simulink model "gm_sobelFilter2024a"  (R2024b)
settings: Solver=FixedStepDiscrete  StartTime=0.0  StopTime=2  FixedStep=2.77039007092199e-06  RelTol=1e-3
undefined symbols (not defined in the file or in its folder): gray, R
libraries: hdlsllib x12, visionhdlio x4, visionsources x2
(part 1 of 2)
Description:
  | Sobel Edge Detection Using the MATLAB(R) Function Block
  | This example shows how to use HDL Coder(TM) to check,
  | generate, and verify HDL code for a Sobel Edge Detection
  | block built using the MATLAB Function block.
settings Model: Creator=The MathWorks, Inc.  LastModifiedBy=avate
settings SolverCC: AlgebraicLoopSolver=TrustRegion
settings DataIOCC: LimitDataPoints=on  SaveFormat=Array  SignalLogging=off  ReturnWorkspaceOutputs=off
settings OptimizationCC: BlockReduction=off  ConditionallyExecuteInputs=off  DefaultParameterBehavior=Inlined  ExpressionDepthLimit=2147483647  InitFltsAndDblsToZero=on  EfficientMapNaN2IntZero=off  LifeSpan=inf
settings DebuggingCC: AlgebraicLoopMsg=error  SaveWithParameterizedLinksMsg=none  MergeDetectMultiDrivingBlocksExec=none  SignalResolutionControl=TryResolveAllWithWarning  InheritedTsInSrcMsg=none  MultiTaskDSMMsg=warning  MultiTaskCondExecSysMsg=none  SingleTaskRateTransMsg=error  IntegerOverflowMsg=none  ParameterPrecisionLossMsg=none  FcnCallInpInsideContextMsg=warning  UnconnectedInputMsg=warning  UnconnectedOutputMsg=warning  UnconnectedLineMsg=warning  AllowSymbolicDim=off  StateNameClashWarn=warning  StrictBusMsg=ErrorOnBusTreatedAsVector  SFUnexpectedBacktrackingDiag=warning  SFNoUnconditionalDefaultTransitionDiag=warning  SFExecutionAtInitializationDiag=none  IntegerSaturationMsg=none  ArithmeticOperatorsInVariantConditions=warning
settings HardwareCC: ProdBitPerPointer=32  ProdBitPerSizeT=32  ProdBitPerPtrDiffT=32  ProdLargestAtomicFloat=None  ProdIntDivRoundTo=Undefined  ProdEndianess=Unspecified  ProdWordSize=32  ProdHWDeviceType=ASIC/FPGA  TargetHWDeviceType=32-bit Generic  ProdEqTarget=off
settings ModelReferenceCC: EnableRefExpFcnMdlSchedulingChecks=on  PropagateSignalLabelsOutOfModel=off
settings SFSimCC: SimUseLocalCustomCode=off  CustomCodeUndefinedFunction=UseInterfaceOnly
settings RTWCC: RTWUseLocalCustomCode=off  GPUComputeCapability=3.5  DLArmComputeVersion=19.05
settings CodeAppCC: StateflowObjectComments=on
settings GRTTargetCC: TargetFcnLib=ansi_tfl_tmw.mat  TargetLangStandard=C89/C90 (ANSI)  CombineOutputUpdateFcns=off  GRTInterface=on
settings ConfigComp: CovMetricSettings=dw  CovSaveCumulativeToWorkspaceVar=on  CovSaveSingleToWorkspaceVar=on  CovExternalEMLEnable=off

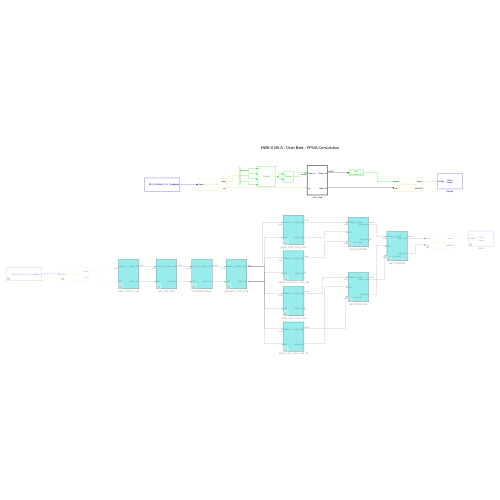
[thumbnail: Simulink's stored preview of the top-level diagram]
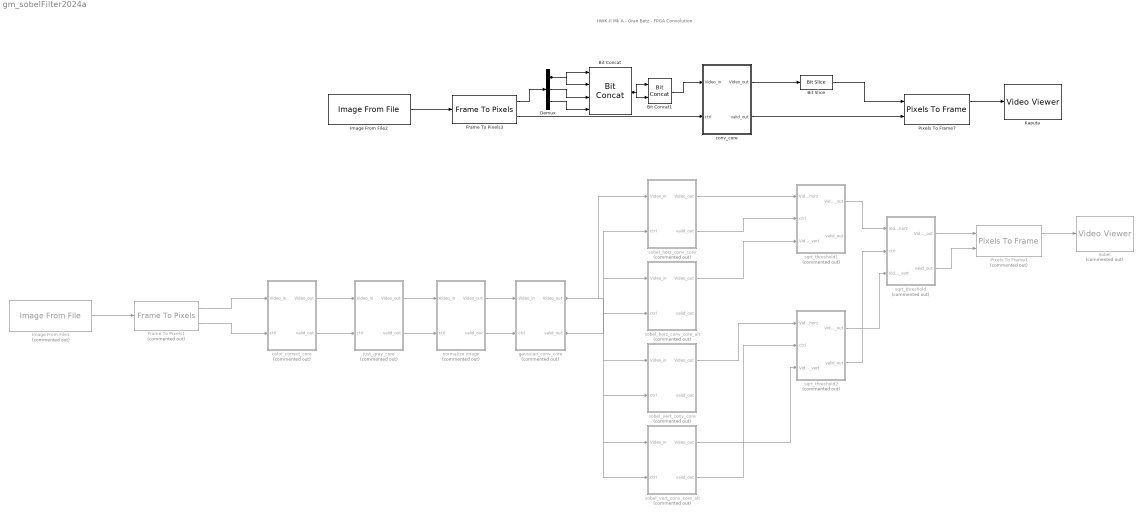
== system gm_sobelFilter2024a ==
  note: HWK-II Mk A - Oran Betz - FPGA Convolution
  Bit Concat : hdlsllib/Logic and Bit Operations/Bit Concat  numInputs=4
  Bit Concat1 : hdlsllib/Logic and Bit Operations/Bit Concat  numInputs=2
  Bit Slice : hdlsllib/Logic and Bit Operations/Bit Slice  lidx=31  ridx=24
  Demux : Demux  Outputs=3
  Frame To Pixels1 : visionhdlio/Frame To Pixels  Commented=on  NumComponents=3  NumPixels=1  VideoFormat=Custom  ActivePixelsPerLine=R  ActiveVideoLines=C  TotalPixelsPerLine=R  TotalVideoLines=C  StartingActiveLine=1  FrontPorch=0  SampleTime=0  VideoFormatCache=Custom  ActivePixelsPerLineCache=R  ActiveVideoLinesCache=C  TotalPixelsPerLineCache=R  TotalVideoLinesCache=C  StartingActiveLineCache=1  FrontPorchCache=0
  Frame To Pixels3 : visionhdlio/Frame To Pixels  NumComponents=3  NumPixels=1  VideoFormat=Custom  ActivePixelsPerLine=R  ActiveVideoLines=C  TotalPixelsPerLine=R  TotalVideoLines=C  StartingActiveLine=1  FrontPorch=0  SampleTime=0  VideoFormatCache=Custom  ActivePixelsPerLineCache=R  ActiveVideoLinesCache=C  TotalPixelsPerLineCache=R  TotalVideoLinesCache=C  StartingActiveLineCache=1  FrontPorchCache=0
  Image From File1 : visionsources/Image From File  Tag=vipblks_nd  Commented=on  FileName=S:\ESD2_Top\ESD2\Final_Proj\Challengers_Sobel\imgs\imgs\BL3_CamLeft_2_5_2.png  Ts=1  imagePorts=One multidimensional signal  OutPortLabels=R|G|B  ImageDataType=Inherit from input image  sdImageDataType=uint(8)  Signed=on  WordLength=16  FractionLengthMode=User-defined  FractionLength=15
  Image From File2 : visionsources/Image From File  Tag=vipblks_nd  FileName=..\imgs\BL3_CamRight_2_5_2.png  Ts=1  imagePorts=One multidimensional signal  OutPortLabels=R|G|B  ImageDataType=Inherit from input image  sdImageDataType=uint(8)  Signed=on  WordLength=16  FractionLengthMode=User-defined  FractionLength=15
  Kaputa : VideoViewer  colormapValue=gray(256)  FigPos=[906 852 825 520]
  Pixels To Frame1 : visionhdlio/Pixels To Frame  Commented=on  NumComponents=1  NumPixels=1  VideoFormat=Custom  ActivePixelsPerLine=R  ActiveVideoLines=C  TotalPixelsPerLine=R  TotalVideoLines=C  VideoFormatCache=Custom  ActivePixelsPerLineCache=R  ActiveVideoLinesCache=C  TotalPixelsPerLineCache=R  TotalVideoLinesCache=C
  Pixels To Frame7 : visionhdlio/Pixels To Frame  NumComponents=1  NumPixels=1  VideoFormat=Custom  ActivePixelsPerLine=R  ActiveVideoLines=C  TotalPixelsPerLine=R  TotalVideoLines=C  VideoFormatCache=Custom  ActivePixelsPerLineCache=R  ActiveVideoLinesCache=C  TotalPixelsPerLineCache=R  TotalVideoLinesCache=C
  Sobel : VideoViewer  Commented=on  colormapValue=gray(256)  FigPos=[2938 790 825 520]
  color_correct_core : Subsystem  Commented=on  TreatAsAtomicUnit=on
  conv_core : Subsystem  TreatAsAtomicUnit=on
  gaussian_conv_core : Subsystem  Commented=on  TreatAsAtomicUnit=on
  just_gray_core : Subsystem  Commented=on  TreatAsAtomicUnit=on
  normalize image : Subsystem  Commented=on  TreatAsAtomicUnit=on
  sobel_horz_conv_core : Subsystem  Commented=on  TreatAsAtomicUnit=on
  sobel_horz_conv_core_alt : Subsystem  Commented=on  TreatAsAtomicUnit=on
  sobel_vert_conv_core : Subsystem  Commented=on  TreatAsAtomicUnit=on
  sobel_vert_conv_core_alt : Subsystem  Commented=on  TreatAsAtomicUnit=on
  sqrt_threshold : Subsystem  Commented=on  TreatAsAtomicUnit=on
  sqrt_threshold1 : Subsystem  Commented=on  TreatAsAtomicUnit=on
  sqrt_threshold2 : Subsystem  Commented=on  TreatAsAtomicUnit=on
  wires:
  Bit Concat/1 -> Bit Concat1/1, Bit Concat1/2
  Bit Concat1/1 -> conv_core/1(Video_in)
  Demux/1 -> Bit Concat/2, Bit Concat/1
  Demux/2 -> Bit Concat/3
  Demux/3 -> Bit Concat/4
  Frame To Pixels1/2 -> color_correct_core/2(ctrl)
  Frame To Pixels1/1 -> color_correct_core/1(Video_in)
  color_correct_core/2(valid_out) -> just_gray_core/2(ctrl)
  color_correct_core/1(Video_out) -> just_gray_core/1(Video_in)
  sobel_vert_conv_core_alt/2(valid_out) -> sqrt_threshold2/2(ctrl)
  sobel_vert_conv_core_alt/1(Video_out) -> sqrt_threshold2/3(Video_in_vert)
  sobel_vert_conv_core/1(Video_out) -> sqrt_threshold2/1(Video_in_horz)
  sobel_horz_conv_core/2(valid_out) -> sqrt_threshold1/2(ctrl)
  sobel_horz_conv_core/1(Video_out) -> sqrt_threshold1/1(Video_in_horz)
  sobel_horz_conv_core_alt/1(Video_out) -> sqrt_threshold1/3(Video_in_vert)
  sqrt_threshold2/2(valid_out) -> sqrt_threshold/2(ctrl)
  sqrt_threshold2/1(Video_out) -> sqrt_threshold/3(Video_in_vert)
  sqrt_threshold1/1(Video_out) -> sqrt_threshold/1(Video_in_horz)
  sqrt_threshold/2(valid_out) -> Pixels To Frame1/2
  sqrt_threshold/1(Video_out) -> Pixels To Frame1/1
  normalize image/2(valid_out) -> gaussian_conv_core/2(ctrl)
  gaussian_conv_core/2(valid_out) -> sobel_horz_conv_core/2(ctrl), sobel_horz_conv_core_alt/2(ctrl), sobel_vert_conv_core_alt/2(ctrl), sobel_vert_conv_core/2(ctrl)
  just_gray_core/1(Video_out) -> normalize image/1(Video_in)
  gaussian_conv_core/1(Video_out) -> sobel_horz_conv_core/1(Video_in), sobel_horz_conv_core_alt/1(Video_in), sobel_vert_conv_core/1(Video_in), sobel_vert_conv_core_alt/1(Video_in)
  just_gray_core/2(valid_out) -> normalize image/2(ctrl)
  normalize image/1(Video_out) -> gaussian_conv_core/1(Video_in)
  Pixels To Frame1/1 -> Sobel/1
  Image From File1/1 -> Frame To Pixels1/1
  Bit Slice/1 -> Pixels To Frame7/1
  conv_core/1(Video_out) -> Bit Slice/1
  conv_core/2(valid_out) -> Pixels To Frame7/2
  Frame To Pixels3/2 -> conv_core/2(ctrl)
  Pixels To Frame7/1 -> Kaputa/1
  Image From File2/1 -> Frame To Pixels3/1
  Frame To Pixels3/1 -> Demux/1

== system gm_sobelFilter2024a/color_correct_core ==
  Video_in : Inport  OutDataTypeStr=uint8
  ctrl : Inport  Port=2
  Bus Selector : BusSelector  OutputSignals=valid
  Subsystem1 : Subsystem
  Video_out : Outport  OutDataTypeStr=uint8  VectorParamsAs1DForOutWhenUnconnected=off
  valid_out : Outport  Port=2  VectorParamsAs1DForOutWhenUnconnected=off
  wires:
  ctrl/1 -> Bus Selector/1, valid_out/1
  Subsystem1/1(Video_out) -> Video_out/1
  Bus Selector/1 -> Subsystem1/Enable  "<valid>"
  Video_in/1 -> Subsystem1/1(channel_in)

== system gm_sobelFilter2024a/conv_core ==
  Video_in : Inport  OutDataTypeStr=fixdt(0, 64, 0)  PortDimensions=1  SampleTime=2.77039007092199e-06
  ctrl : Inport  Port=2
  Bit Concat : hdlsllib/Logic and Bit Operations/Bit Concat  numInputs=8
  Bit Slice : hdlsllib/Logic and Bit Operations/Bit Slice  lidx=double(31)  ridx=double(0)
  color_correct_core : Subsystem
  gaussian_conv_core : Subsystem
  just_gray_core : Subsystem
  normalize image : Subsystem
  sobel_horz_conv_core : Subsystem
  sobel_horz_conv_core_alt : Subsystem
  sobel_vert_conv_core : Subsystem
  sobel_vert_conv_core_alt : Subsystem
  sqrt_threshold : Subsystem
  sqrt_threshold1 : Subsystem
  sqrt_threshold2 : Subsystem
  Video_out : Outport  OutDataTypeStr=uint64  SampleTime=2.77039007092199e-06  VectorParamsAs1DForOutWhenUnconnected=off
  valid_out : Outport  Port=2  VectorParamsAs1DForOutWhenUnconnected=off
  wires:
  normalize image/1(Video_out) -> gaussian_conv_core/1(Video_in)
  Video_in/1 -> Bit Slice/1
  sqrt_threshold1/1(Video_out) -> sqrt_threshold/1(Video_in_horz)
  Bit Slice/1 -> color_correct_core/1(Video_in)
  ctrl/1 -> color_correct_core/2(ctrl)
  color_correct_core/1(Video_out) -> just_gray_core/1(Video_in)
  just_gray_core/2(valid_out) -> normalize image/2(ctrl)
  color_correct_core/2(valid_out) -> just_gray_core/2(ctrl)
  just_gray_core/1(Video_out) -> normalize image/1(Video_in)
  Bit Concat/1 -> Video_out/1
  gaussian_conv_core/2(valid_out) -> sobel_vert_conv_core_alt/2(ctrl), sobel_horz_conv_core_alt/2(ctrl), sobel_vert_conv_core/2(ctrl), sobel_horz_conv_core/2(ctrl)
  normalize image/2(valid_out) -> gaussian_conv_core/2(ctrl)
  gaussian_conv_core/1(Video_out) -> sobel_vert_conv_core/1(Video_in), sobel_vert_conv_core_alt/1(Video_in), sobel_horz_conv_core_alt/1(Video_in), sobel_horz_conv_core/1(Video_in)
  sobel_horz_conv_core/1(Video_out) -> sqrt_threshold1/1(Video_in_horz)
  sobel_horz_conv_core/2(valid_out) -> sqrt_threshold1/2(ctrl)
  sobel_horz_conv_core_alt/1(Video_out) -> sqrt_threshold1/3(Video_in_vert)
  sobel_vert_conv_core/1(Video_out) -> sqrt_threshold2/1(Video_in_horz)
  sobel_vert_conv_core_alt/1(Video_out) -> sqrt_threshold2/3(Video_in_vert)
  sobel_vert_conv_core_alt/2(valid_out) -> sqrt_threshold2/2(ctrl)
  sqrt_threshold2/1(Video_out) -> sqrt_threshold/3(Video_in_vert)
  sqrt_threshold2/2(valid_out) -> sqrt_threshold/2(ctrl)
  sqrt_threshold/1(Video_out) -> Bit Concat/7, Bit Concat/6, Bit Concat/5, Bit Concat/8, Bit Concat/3, Bit Concat/1, Bit Concat/2, Bit Concat/4
  sqrt_threshold/2(valid_out) -> valid_out/1

== system gm_sobelFilter2024a/gaussian_conv_core ==
  note: Coefficients Constants Block
  Video_in : Inport  OutDataTypeStr=uint8
  ctrl : Inport  Port=2
  Bus Selector : BusSelector  OutputSignals=valid
  Constant : Constant  Value=[1/16 1/8 1/16; 1/8 1/4 1/8; 1/16 1/8 1/16];  OutDataTypeStr=fixdt(1,16,12)  SampleTime=-1
  Delay1 : Delay  InitialCondition=0
  Reshape : Reshape
  Subsystem1 : Subsystem
  Transpose : Math  Operator=transpose
  Video_out : Outport  OutDataTypeStr=uint8  VectorParamsAs1DForOutWhenUnconnected=off
  valid_out : Outport  Port=2  VectorParamsAs1DForOutWhenUnconnected=off
  wires:
  Constant/1 -> Transpose/1
  Transpose/1 -> Reshape/1
  Delay1/1 -> valid_out/1
  Reshape/1 -> Subsystem1/2(coeffs)
  Subsystem1/1(Video_out) -> Video_out/1
  Bus Selector/1 -> Subsystem1/Enable  "<valid>"
  ctrl/1 -> Delay1/1, Bus Selector/1
  Video_in/1 -> Subsystem1/1(channel_in)

== system gm_sobelFilter2024a/just_gray_core ==
  Video_in : Inport  OutDataTypeStr=uint8
  ctrl : Inport  Port=2
  Bus Selector : BusSelector  OutputSignals=valid
  Subsystem1 : Subsystem
  Video_out : Outport  OutDataTypeStr=uint8  VectorParamsAs1DForOutWhenUnconnected=off
  valid_out : Outport  Port=2  VectorParamsAs1DForOutWhenUnconnected=off
  wires:
  ctrl/1 -> Bus Selector/1, valid_out/1
  Subsystem1/1(Video_out) -> Video_out/1
  Bus Selector/1 -> Subsystem1/Enable  "<valid>"
  Video_in/1 -> Subsystem1/1(channel_in)

== system gm_sobelFilter2024a/normalize image ==
  Video_in : Inport  OutDataTypeStr=uint8
  ctrl : Inport  Port=2
  Bus Selector : BusSelector  OutputSignals=valid
  Delay3 : Delay  DelayLength=4  InitialCondition=0
  Subsystem1 : Subsystem
  Video_out : Outport  OutDataTypeStr=uint8  VectorParamsAs1DForOutWhenUnconnected=off
  valid_out : Outport  Port=2  VectorParamsAs1DForOutWhenUnconnected=off
  wires:
  Delay3/1 -> valid_out/1
  ctrl/1 -> Bus Selector/1, Delay3/1
  Subsystem1/1(Video_out) -> Video_out/1
  Bus Selector/1 -> Subsystem1/Enable  "<valid>"
  Video_in/1 -> Subsystem1/1(channel_in)

== system gm_sobelFilter2024a/sobel_horz_conv_core ==
  note: Coefficients Constants Block
  Video_in : Inport  OutDataTypeStr=uint8
  ctrl : Inport  Port=2
  Bus Selector : BusSelector  OutputSignals=valid
  Constant : Constant  Value=[1 0 -1; 2 0 -2; 1 0 -1];  OutDataTypeStr=fixdt(1,16,12)  SampleTime=-1
  Delay1 : Delay  InitialCondition=0
  Reshape : Reshape
  Subsystem1 : Subsystem
  Transpose : Math  Operator=transpose
  Video_out : Outport  OutDataTypeStr=uint8  VectorParamsAs1DForOutWhenUnconnected=off
  valid_out : Outport  Port=2  VectorParamsAs1DForOutWhenUnconnected=off
  wires:
  Constant/1 -> Transpose/1
  Transpose/1 -> Reshape/1
  Delay1/1 -> valid_out/1
  Reshape/1 -> Subsystem1/2(coeffs)
  Subsystem1/1(Video_out) -> Video_out/1
  Bus Selector/1 -> Subsystem1/Enable  "<valid>"
  ctrl/1 -> Delay1/1, Bus Selector/1
  Video_in/1 -> Subsystem1/1(channel_in)

== system gm_sobelFilter2024a/sobel_horz_conv_core_alt ==
  note: Coefficients Constants Block
  Video_in : Inport  OutDataTypeStr=uint8
  ctrl : Inport  Port=2
  Bus Selector : BusSelector  OutputSignals=valid
  Constant : Constant  Value=[-1 0 1; -2 0 2; -1 0 1];  OutDataTypeStr=fixdt(1,16,12)  SampleTime=-1
  Delay1 : Delay  InitialCondition=0
  Reshape : Reshape
  Subsystem1 : Subsystem
  Transpose : Math  Operator=transpose
  Video_out : Outport  OutDataTypeStr=uint8  VectorParamsAs1DForOutWhenUnconnected=off
  valid_out : Outport  Port=2  VectorParamsAs1DForOutWhenUnconnected=off
  wires:
  Constant/1 -> Transpose/1
  Transpose/1 -> Reshape/1
  Delay1/1 -> valid_out/1
  Reshape/1 -> Subsystem1/2(coeffs)
  Subsystem1/1(Video_out) -> Video_out/1
  Bus Selector/1 -> Subsystem1/Enable  "<valid>"
  ctrl/1 -> Delay1/1, Bus Selector/1
  Video_in/1 -> Subsystem1/1(channel_in)

== system gm_sobelFilter2024a/sobel_vert_conv_core ==
  note: Coefficients Constants Block
  Video_in : Inport  OutDataTypeStr=uint8
  ctrl : Inport  Port=2
  Bus Selector : BusSelector  OutputSignals=valid
  Constant : Constant  Value=|  OutDataTypeStr=fixdt(1,16,12)  SampleTime=-1
      | [1 2 1;  0 0 0;
      | -1 -2 -1];
  Delay1 : Delay  InitialCondition=0
  Reshape : Reshape
  Subsystem1 : Subsystem
  Transpose : Math  Operator=transpose
  Video_out : Outport  OutDataTypeStr=uint8  VectorParamsAs1DForOutWhenUnconnected=off
  valid_out : Outport  Port=2  VectorParamsAs1DForOutWhenUnconnected=off
  wires:
  Constant/1 -> Transpose/1
  Transpose/1 -> Reshape/1
  Delay1/1 -> valid_out/1
  Reshape/1 -> Subsystem1/2(coeffs)
  Subsystem1/1(Video_out) -> Video_out/1
  Bus Selector/1 -> Subsystem1/Enable  "<valid>"
  ctrl/1 -> Delay1/1, Bus Selector/1
  Video_in/1 -> Subsystem1/1(channel_in)

== system gm_sobelFilter2024a/sobel_vert_conv_core_alt ==
  note: Coefficients Constants Block
  Video_in : Inport  OutDataTypeStr=uint8
  ctrl : Inport  Port=2
  Bus Selector : BusSelector  OutputSignals=valid
  Constant : Constant  Value=|  OutDataTypeStr=fixdt(1,16,12)  SampleTime=-1
      | [-1 -2 -1;  0 0 0;
      | 1 2 1];
  Delay1 : Delay  InitialCondition=0
  Reshape : Reshape
  Subsystem1 : Subsystem
  Transpose : Math  Operator=transpose
  Video_out : Outport  OutDataTypeStr=uint8  VectorParamsAs1DForOutWhenUnconnected=off
  valid_out : Outport  Port=2  VectorParamsAs1DForOutWhenUnconnected=off
  wires:
  Constant/1 -> Transpose/1
  Transpose/1 -> Reshape/1
  Delay1/1 -> valid_out/1
  Reshape/1 -> Subsystem1/2(coeffs)
  Subsystem1/1(Video_out) -> Video_out/1
  Bus Selector/1 -> Subsystem1/Enable  "<valid>"
  ctrl/1 -> Delay1/1, Bus Selector/1
  Video_in/1 -> Subsystem1/1(channel_in)

== system gm_sobelFilter2024a/sqrt_threshold ==
  note: Coefficients Constants Block
  Video_in_horz : Inport  OutDataTypeStr=uint8
  ctrl : Inport  Port=2
  Video_in_vert : Inport  Port=3  OutDataTypeStr=uint8
  Bus Selector : BusSelector  OutputSignals=valid
  Constant : Constant  Value=|  OutDataTypeStr=fixdt(1,16,12)  SampleTime=-1
      | [1 2 1;  0 0 0;
      | -1 -2 -2];
  Delay1 : Delay  DelayLength=4  InitialCondition=0
  Reshape : Reshape
  Subsystem2 : Subsystem
  Transpose : Math  Operator=transpose
  Video_out : Outport  OutDataTypeStr=uint8  VectorParamsAs1DForOutWhenUnconnected=off
  valid_out : Outport  Port=2  VectorParamsAs1DForOutWhenUnconnected=off
  wires:
  Video_in_vert/1 -> Subsystem2/2(channel_in_vert)
  Constant/1 -> Transpose/1
  Transpose/1 -> Reshape/1
  Delay1/1 -> valid_out/1
  Reshape/1 -> Subsystem2/3(coeffs)
  Subsystem2/1(Video_out) -> Video_out/1
  Bus Selector/1 -> Subsystem2/Enable  "<valid>"
  ctrl/1 -> Delay1/1, Bus Selector/1
  Video_in_horz/1 -> Subsystem2/1(channel_horz)

== system gm_sobelFilter2024a/sqrt_threshold1 ==
  note: Coefficients Constants Block
  Video_in_horz : Inport  OutDataTypeStr=uint8
  ctrl : Inport  Port=2
  Video_in_vert : Inport  Port=3  OutDataTypeStr=uint8
  Bus Selector : BusSelector  OutputSignals=valid
  Constant : Constant  Value=|  OutDataTypeStr=fixdt(1,16,12)  SampleTime=-1
      | [1 2 1;  0 0 0;
      | -1 -2 -2];
  Delay1 : Delay  DelayLength=4  InitialCondition=0
  Reshape : Reshape
  Subsystem2 : Subsystem
  Transpose : Math  Operator=transpose
  Video_out : Outport  OutDataTypeStr=uint8  VectorParamsAs1DForOutWhenUnconnected=off
  valid_out : Outport  Port=2  VectorParamsAs1DForOutWhenUnconnected=off
  wires:
  Video_in_vert/1 -> Subsystem2/2(channel_in_vert)
  Constant/1 -> Transpose/1
  Transpose/1 -> Reshape/1
  Delay1/1 -> valid_out/1
  Reshape/1 -> Subsystem2/3(coeffs)
  Subsystem2/1(Video_out) -> Video_out/1
  Bus Selector/1 -> Subsystem2/Enable  "<valid>"
  ctrl/1 -> Delay1/1, Bus Selector/1
  Video_in_horz/1 -> Subsystem2/1(channel_horz)

== system gm_sobelFilter2024a/sqrt_threshold2 ==
  note: Coefficients Constants Block
  Video_in_horz : Inport  OutDataTypeStr=uint8
  ctrl : Inport  Port=2
  Video_in_vert : Inport  Port=3  OutDataTypeStr=uint8
  Bus Selector : BusSelector  OutputSignals=valid
  Constant : Constant  Value=|  OutDataTypeStr=fixdt(1,16,12)  SampleTime=-1
      | [1 2 1;  0 0 0;
      | -1 -2 -2];
  Delay1 : Delay  DelayLength=4  InitialCondition=0
  Reshape : Reshape
  Subsystem2 : Subsystem
  Transpose : Math  Operator=transpose
  Video_out : Outport  OutDataTypeStr=uint8  VectorParamsAs1DForOutWhenUnconnected=off
  valid_out : Outport  Port=2  VectorParamsAs1DForOutWhenUnconnected=off
  wires:
  Video_in_vert/1 -> Subsystem2/2(channel_in_vert)
  Constant/1 -> Transpose/1
  Transpose/1 -> Reshape/1
  Delay1/1 -> valid_out/1
  Reshape/1 -> Subsystem2/3(coeffs)
  Subsystem2/1(Video_out) -> Video_out/1
  Bus Selector/1 -> Subsystem2/Enable  "<valid>"
  ctrl/1 -> Delay1/1, Bus Selector/1
  Video_in_horz/1 -> Subsystem2/1(channel_horz)

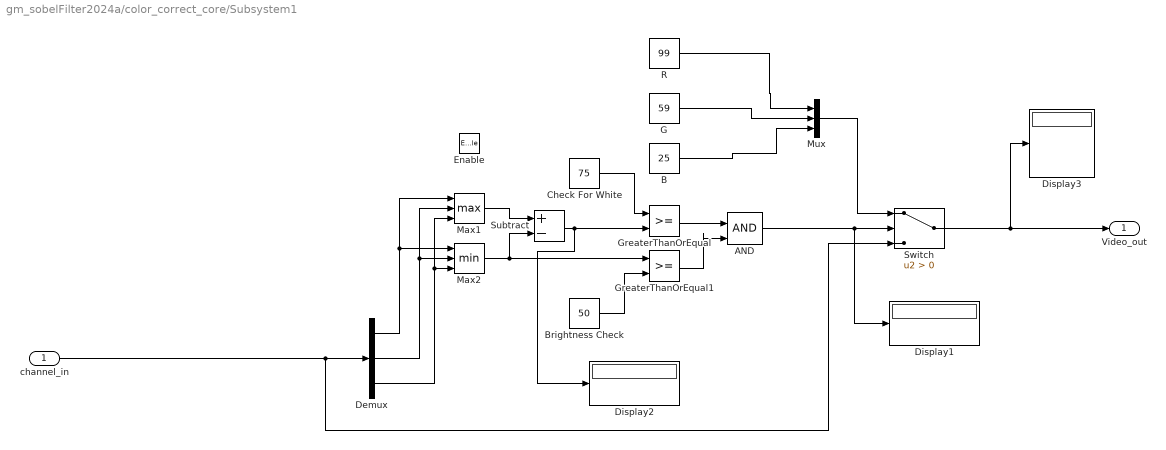
== system gm_sobelFilter2024a/color_correct_core/Subsystem1 ==
  channel_in : Inport  OutDataTypeStr=uint8
  Enable : EnablePort
  AND : Logic  IconShape=distinctive  AllPortsSameDT=off  OutDataTypeStr=boolean
  B : Constant  Value=25  OutDataTypeStr=uint8
  Brightness Check : Constant  Value=50  OutDataTypeStr=uint8
  Check For White : Constant  Value=75  OutDataTypeStr=uint8
  Demux : Demux  Outputs=3
  Display1 : Display
      settings: Format=binary (Stored Integer)
  Display2 : Display
      settings: Format=binary (Stored Integer)
  Display3 : Display
      settings: Format=binary (Stored Integer)
  G : Constant  Value=59  OutDataTypeStr=uint8
  GreaterThanOrEqual : RelationalOperator  OutDataTypeStr=boolean  RndMeth=Simplest  InputSameDT=off
  GreaterThanOrEqual1 : RelationalOperator  OutDataTypeStr=boolean  RndMeth=Simplest  InputSameDT=off
  Max1 : MinMax  Function=max  Inputs=3
  Max2 : MinMax  Inputs=3
  Mux : Mux  Inputs=3
  R : Constant  Value=99  OutDataTypeStr=uint8
  Subtract : Sum  Inputs=+-
  Switch : Switch  Criteria=u2 > Threshold  SaturateOnIntegerOverflow=off  InputSameDT=off
  Video_out : Outport  OutDataTypeStr=uint8  InitialOutput=[0]
  wires:
  Mux/1 -> Switch/1
  Switch/1 -> Video_out/1, Display3/1
  B/1 -> Mux/3
  G/1 -> Mux/2
  R/1 -> Mux/1
  AND/1 -> Switch/2, Display1/1
  Subtract/1 -> Display2/1, GreaterThanOrEqual/2
  GreaterThanOrEqual1/1 -> AND/2
  Brightness Check/1 -> GreaterThanOrEqual1/2
  GreaterThanOrEqual/1 -> AND/1
  Check For White/1 -> GreaterThanOrEqual/1
  Max2/1 -> Subtract/2, GreaterThanOrEqual1/1
  Max1/1 -> Subtract/1
  Demux/2 -> Max1/2, Max2/2
  Demux/1 -> Max1/1, Max2/1
  channel_in/1 -> Demux/1, Switch/3
  Demux/3 -> Max1/3, Max2/3

== system gm_sobelFilter2024a/conv_core/color_correct_core ==
  Video_in : Inport  OutDataTypeStr=uint32  PortDimensions=1  SampleTime=2.77039007092199e-06
  ctrl : Inport  Port=2
  Subsystem1 : Subsystem
  bus_selector : BusSelector  OutputSignals=valid
  Video_out : Outport  OutDataTypeStr=uint32  SampleTime=2.77039007092199e-06  VectorParamsAs1DForOutWhenUnconnected=off
  valid_out : Outport  Port=2  VectorParamsAs1DForOutWhenUnconnected=off
  wires:
  ctrl/1 -> bus_selector/1, valid_out/1
  bus_selector/1 -> Subsystem1/Enable  "<valid>"
  Video_in/1 -> Subsystem1/1(channel_in)
  Subsystem1/1(Video_out) -> Video_out/1

== system gm_sobelFilter2024a/conv_core/gaussian_conv_core ==
  note: Coefficients Constants Block
  Video_in : Inport  OutDataTypeStr=uint8  PortDimensions=1  SampleTime=2.77039007092199e-06
  ctrl : Inport  Port=2
  Constant : Constant  Value=[0.0625;0.125;0.0625;0.125;0.25;0.125;0.0625;0.125;0.0625]  OutDataTypeStr=fixdt(1, 16, 12)  SampleTime=2.77039007092199e-06
  Delay1 : Delay  DelayLength=double(2)  InitialCondition=0  SampleTime=2.77039007092199e-06
  Reshape : Reshape  OutputDimensions=[9]
  Subsystem1 : Subsystem
  Transpose : Math  Operator=transpose  OutDataTypeStr=fixdt(1, 16, 12)
  bus_selector : BusSelector  OutputSignals=valid
  t : Reshape  OutputDimensionality=Customize  OutputDimensions=[3,3]
  Video_out : Outport  OutDataTypeStr=uint8  SampleTime=2.77039007092199e-06  VectorParamsAs1DForOutWhenUnconnected=off
  valid_out : Outport  Port=2  VectorParamsAs1DForOutWhenUnconnected=off
  wires:
  Constant/1 -> t/1
  Reshape/1 -> Subsystem1/2(coeffs)
  t/1 -> Transpose/1
  Transpose/1 -> Reshape/1
  bus_selector/1 -> Subsystem1/Enable  "<valid>"
  Delay1/1 -> valid_out/1
  ctrl/1 -> bus_selector/1, Delay1/1
  Video_in/1 -> Subsystem1/1(channel_in)
  Subsystem1/1(Video_out) -> Video_out/1

== system gm_sobelFilter2024a/conv_core/just_gray_core ==
  Video_in : Inport  OutDataTypeStr=uint32  PortDimensions=1  SampleTime=2.77039007092199e-06
  ctrl : Inport  Port=2
  Subsystem1 : Subsystem
  bus_selector : BusSelector  OutputSignals=valid
  Video_out : Outport  OutDataTypeStr=uint8  SampleTime=2.77039007092199e-06  VectorParamsAs1DForOutWhenUnconnected=off
  valid_out : Outport  Port=2  VectorParamsAs1DForOutWhenUnconnected=off
  wires:
  ctrl/1 -> bus_selector/1, valid_out/1
  bus_selector/1 -> Subsystem1/Enable  "<valid>"
  Subsystem1/1(Video_out) -> Video_out/1
  Video_in/1 -> Subsystem1/1(channel_in)

== system gm_sobelFilter2024a/conv_core/normalize image ==
  Video_in : Inport  OutDataTypeStr=uint8  PortDimensions=1  SampleTime=2.77039007092199e-06
  ctrl : Inport  Port=2
  Delay3 : Delay  DelayLength=double(4)  InitialCondition=0  SampleTime=2.77039007092199e-06
  Subsystem1 : Subsystem
  bus_selector : BusSelector  OutputSignals=valid
  Video_out : Outport  OutDataTypeStr=uint8  SampleTime=2.77039007092199e-06  VectorParamsAs1DForOutWhenUnconnected=off
  valid_out : Outport  Port=2  VectorParamsAs1DForOutWhenUnconnected=off
  wires:
  Subsystem1/1(Video_out) -> Video_out/1
  Delay3/1 -> valid_out/1
  ctrl/1 -> bus_selector/1, Delay3/1
  bus_selector/1 -> Subsystem1/Enable  "<valid>"
  Video_in/1 -> Subsystem1/1(channel_in)

== system gm_sobelFilter2024a/conv_core/sobel_horz_conv_core ==
  note: Coefficients Constants Block
  Video_in : Inport  OutDataTypeStr=uint8  PortDimensions=1  SampleTime=2.77039007092199e-06
  ctrl : Inport  Port=2
  Constant : Constant  Value=[1;2;1;0;0;0;-1;-2;-1]  OutDataTypeStr=fixdt(1, 16, 12)  SampleTime=2.77039007092199e-06
  Delay1 : Delay  DelayLength=double(2)  InitialCondition=0  SampleTime=2.77039007092199e-06
  Reshape : Reshape  OutputDimensions=[9]
  Subsystem1 : Subsystem
  Transpose : Math  Operator=transpose  OutDataTypeStr=fixdt(1, 16, 12)
  bus_selector : BusSelector  OutputSignals=valid
  t : Reshape  OutputDimensionality=Customize  OutputDimensions=[3,3]
  Video_out : Outport  OutDataTypeStr=uint8  SampleTime=2.77039007092199e-06  VectorParamsAs1DForOutWhenUnconnected=off
  valid_out : Outport  Port=2  VectorParamsAs1DForOutWhenUnconnected=off
  wires:
  Reshape/1 -> Subsystem1/2(coeffs)
  t/1 -> Transpose/1
  bus_selector/1 -> Subsystem1/Enable  "<valid>"
  ctrl/1 -> bus_selector/1, Delay1/1
  Constant/1 -> t/1
  Transpose/1 -> Reshape/1
  Video_in/1 -> Subsystem1/1(channel_in)
  Delay1/1 -> valid_out/1
  Subsystem1/1(Video_out) -> Video_out/1

== system gm_sobelFilter2024a/conv_core/sobel_horz_conv_core_alt ==
  note: Coefficients Constants Block
  Video_in : Inport  OutDataTypeStr=uint8  PortDimensions=1  SampleTime=2.77039007092199e-06
  ctrl : Inport  Port=2
  Constant : Constant  Value=[-1;-2;-1;0;0;0;1;2;1]  OutDataTypeStr=fixdt(1, 16, 12)  SampleTime=2.77039007092199e-06
  Reshape : Reshape  OutputDimensions=[9]
  Subsystem1 : Subsystem
  Transpose : Math  Operator=transpose  OutDataTypeStr=fixdt(1, 16, 12)
  bus_selector : BusSelector  OutputSignals=valid
  t : Reshape  OutputDimensionality=Customize  OutputDimensions=[3,3]
  Video_out : Outport  OutDataTypeStr=uint8  SampleTime=2.77039007092199e-06  VectorParamsAs1DForOutWhenUnconnected=off
  wires:
  Video_in/1 -> Subsystem1/1(channel_in)
  Constant/1 -> t/1
  Transpose/1 -> Reshape/1
  t/1 -> Transpose/1
  Reshape/1 -> Subsystem1/2(coeffs)
  bus_selector/1 -> Subsystem1/Enable  "<valid>"
  ctrl/1 -> bus_selector/1
  Subsystem1/1(Video_out) -> Video_out/1

== system gm_sobelFilter2024a/conv_core/sobel_vert_conv_core ==
  note: Coefficients Constants Block
  Video_in : Inport  OutDataTypeStr=uint8  PortDimensions=1  SampleTime=2.77039007092199e-06
  ctrl : Inport  Port=2
  Constant : Constant  Value=[1;0;-1;2;0;-2;1;0;-1]  OutDataTypeStr=fixdt(1, 16, 12)  SampleTime=2.77039007092199e-06
  Reshape : Reshape  OutputDimensions=[9]
  Subsystem1 : Subsystem
  Transpose : Math  Operator=transpose  OutDataTypeStr=fixdt(1, 16, 12)
  bus_selector : BusSelector  OutputSignals=valid
  t : Reshape  OutputDimensionality=Customize  OutputDimensions=[3,3]
  Video_out : Outport  OutDataTypeStr=uint8  SampleTime=2.77039007092199e-06  VectorParamsAs1DForOutWhenUnconnected=off
  wires:
  Reshape/1 -> Subsystem1/2(coeffs)
  bus_selector/1 -> Subsystem1/Enable  "<valid>"
  t/1 -> Transpose/1
  Constant/1 -> t/1
  Subsystem1/1(Video_out) -> Video_out/1
  Video_in/1 -> Subsystem1/1(channel_in)
  ctrl/1 -> bus_selector/1
  Transpose/1 -> Reshape/1

== system gm_sobelFilter2024a/conv_core/sobel_vert_conv_core_alt ==
  note: Coefficients Constants Block
  Video_in : Inport  OutDataTypeStr=uint8  PortDimensions=1  SampleTime=2.77039007092199e-06
  ctrl : Inport  Port=2
  Constant : Constant  Value=[-1;0;1;-2;0;2;-1;0;1]  OutDataTypeStr=fixdt(1, 16, 12)  SampleTime=2.77039007092199e-06
  Delay1 : Delay  DelayLength=double(2)  InitialCondition=0  SampleTime=2.77039007092199e-06
  Reshape : Reshape  OutputDimensions=[9]
  Subsystem1 : Subsystem
  Transpose : Math  Operator=transpose  OutDataTypeStr=fixdt(1, 16, 12)
  bus_selector : BusSelector  OutputSignals=valid
  t : Reshape  OutputDimensionality=Customize  OutputDimensions=[3,3]
  Video_out : Outport  OutDataTypeStr=uint8  SampleTime=2.77039007092199e-06  VectorParamsAs1DForOutWhenUnconnected=off
  valid_out : Outport  Port=2  VectorParamsAs1DForOutWhenUnconnected=off
  wires:
  Constant/1 -> t/1
  Reshape/1 -> Subsystem1/2(coeffs)
  Transpose/1 -> Reshape/1
  t/1 -> Transpose/1
  ctrl/1 -> bus_selector/1, Delay1/1
  bus_selector/1 -> Subsystem1/Enable  "<valid>"
  Delay1/1 -> valid_out/1
  Video_in/1 -> Subsystem1/1(channel_in)
  Subsystem1/1(Video_out) -> Video_out/1

== system gm_sobelFilter2024a/conv_core/sqrt_threshold ==
  note: Coefficients Constants Block
  Video_in_horz : Inport  OutDataTypeStr=uint8  PortDimensions=1  SampleTime=2.77039007092199e-06
  ctrl : Inport  Port=2
  Video_in_vert : Inport  Port=3  OutDataTypeStr=uint8  PortDimensions=1  SampleTime=2.77039007092199e-06
  Delay1 : Delay  DelayLength=double(4)  InitialCondition=0  SampleTime=2.77039007092199e-06
  Subsystem2 : Subsystem
  bus_selector : BusSelector  OutputSignals=valid
  Video_out : Outport  OutDataTypeStr=uint8  SampleTime=2.77039007092199e-06  VectorParamsAs1DForOutWhenUnconnected=off
  valid_out : Outport  Port=2  VectorParamsAs1DForOutWhenUnconnected=off
  wires:
  bus_selector/1 -> Subsystem2/Enable  "<valid>"
  ctrl/1 -> bus_selector/1, Delay1/1
  Delay1/1 -> valid_out/1
  Video_in_horz/1 -> Subsystem2/1(channel_horz)
  Video_in_vert/1 -> Subsystem2/2(channel_in_vert)
  Subsystem2/1(Video_out) -> Video_out/1

== system gm_sobelFilter2024a/conv_core/sqrt_threshold1 ==
  note: Coefficients Constants Block
  Video_in_horz : Inport  OutDataTypeStr=uint8  PortDimensions=1  SampleTime=2.77039007092199e-06
  ctrl : Inport  Port=2
  Video_in_vert : Inport  Port=3  OutDataTypeStr=uint8  PortDimensions=1  SampleTime=2.77039007092199e-06
  Delay1 : Delay  DelayLength=double(4)  InitialCondition=0  SampleTime=2.77039007092199e-06
  Subsystem2 : Subsystem
  bus_selector : BusSelector  OutputSignals=valid
  Video_out : Outport  OutDataTypeStr=uint8  SampleTime=2.77039007092199e-06  VectorParamsAs1DForOutWhenUnconnected=off
  valid_out : Outport  Port=2  VectorParamsAs1DForOutWhenUnconnected=off
  wires:
  Subsystem2/1(Video_out) -> Video_out/1
  Video_in_vert/1 -> Subsystem2/2(channel_in_vert)
  Video_in_horz/1 -> Subsystem2/1(channel_horz)
  Delay1/1 -> valid_out/1
  ctrl/1 -> Delay1/1, bus_selector/1
  bus_selector/1 -> Subsystem2/Enable  "<valid>"

== system gm_sobelFilter2024a/conv_core/sqrt_threshold2 ==
  note: Coefficients Constants Block
  Video_in_horz : Inport  OutDataTypeStr=uint8  PortDimensions=1  SampleTime=2.77039007092199e-06
  ctrl : Inport  Port=2
  Video_in_vert : Inport  Port=3  OutDataTypeStr=uint8  PortDimensions=1  SampleTime=2.77039007092199e-06
  Delay1 : Delay  DelayLength=double(4)  InitialCondition=0  SampleTime=2.77039007092199e-06
  Subsystem2 : Subsystem
  bus_selector : BusSelector  OutputSignals=valid
  Video_out : Outport  OutDataTypeStr=uint8  SampleTime=2.77039007092199e-06  VectorParamsAs1DForOutWhenUnconnected=off
  valid_out : Outport  Port=2  VectorParamsAs1DForOutWhenUnconnected=off
  wires:
  Subsystem2/1(Video_out) -> Video_out/1
  Video_in_vert/1 -> Subsystem2/2(channel_in_vert)
  Video_in_horz/1 -> Subsystem2/1(channel_horz)
  Delay1/1 -> valid_out/1
  ctrl/1 -> Delay1/1, bus_selector/1
  bus_selector/1 -> Subsystem2/Enable  "<valid>"

== system gm_sobelFilter2024a/gaussian_conv_core/Subsystem1 ==
  note: slice out gray
  channel_in : Inport  OutDataTypeStr=uint8
  coeffs : Inport  Port=2
  Enable : EnablePort
  Delay1 : Delay  DelayLength=1  InitialCondition=0
  Delay2 : Delay  DelayLength=1  InitialCondition=0
  Display : Display
      settings: Format=hex (Stored Integer)
  Mux : Mux  Inputs=9
  Product : Product  SaturateOnIntegerOverflow=on
  Sum of Elements : Sum  Inputs=+  OutDataTypeStr=uint8  SaturateOnIntegerOverflow=on
  slicer : Subsystem
  Video_out : Outport  OutDataTypeStr=uint8  InitialOutput=[0]
  wires:
  Delay2/1 -> Video_out/1
  Sum of Elements/1 -> Delay2/1
  Delay1/1 -> Sum of Elements/1
  Product/1 -> Delay1/1
  coeffs/1 -> Display/1, Product/1
  Mux/1 -> Product/2
  slicer/8(out_8) -> Mux/8
  channel_in/1 -> slicer/1(channel_in)
  slicer/2(out_2) -> Mux/2
  slicer/4(out_4) -> Mux/4
  slicer/6(out_6) -> Mux/6
  slicer/3(out_3) -> Mux/3
  slicer/7(out_7) -> Mux/7
  slicer/5(out_5) -> Mux/5
  slicer/9(out_9) -> Mux/9
  slicer/1(out_1) -> Mux/1

== system gm_sobelFilter2024a/just_gray_core/Subsystem1 ==
  note: Grayscale = (R * 0.25) + (G * 0.5) + (B * 0.0625)
  note: slice out gray
  channel_in : Inport  OutDataTypeStr=uint8
  Enable : EnablePort
  Demux : Demux  Outputs=3
  Shift Arithmetic3 : ArithShift  BitShiftNumber=1  BitShiftDirection=Right
  Shift Arithmetic4 : ArithShift  BitShiftNumber=2  BitShiftDirection=Right
  Shift Arithmetic5 : ArithShift  BitShiftNumber=4  BitShiftDirection=Right
  Sum : Sum  Inputs=+++  OutDataTypeStr=uint8
  Video_out : Outport  OutDataTypeStr=uint8  InitialOutput=[0]
  wires:
  Shift Arithmetic5/1 -> Sum/3
  Shift Arithmetic3/1 -> Sum/2
  Demux/1 -> Shift Arithmetic4/1
  Demux/2 -> Shift Arithmetic3/1
  Shift Arithmetic4/1 -> Sum/1
  channel_in/1 -> Demux/1
  Demux/3 -> Shift Arithmetic5/1
  Sum/1 -> Video_out/1

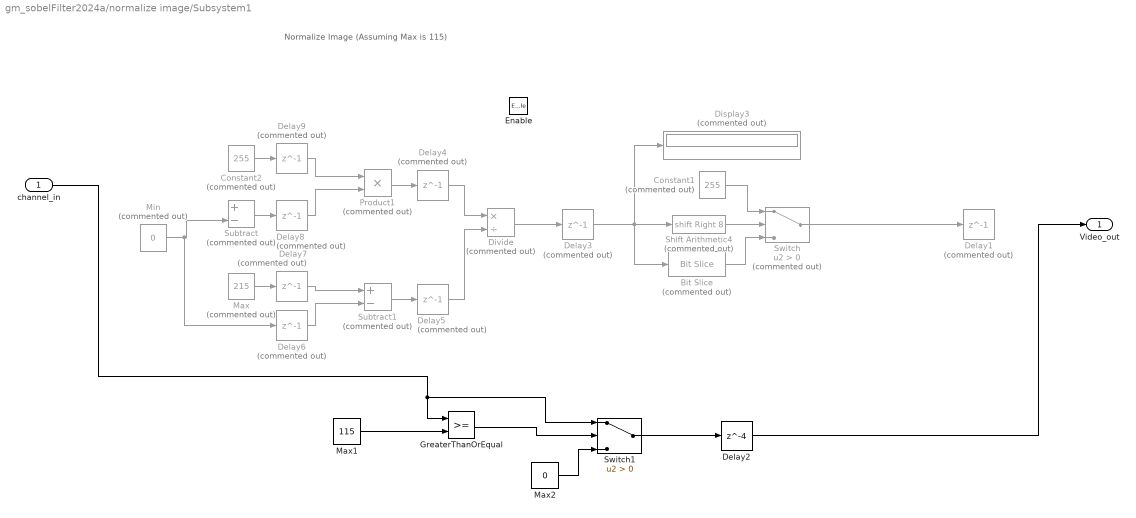
== system gm_sobelFilter2024a/normalize image/Subsystem1 ==
  note: Normalize Image (Assuming Max is 115)
  channel_in : Inport  OutDataTypeStr=uint8
  Enable : EnablePort
  Bit Slice : hdlsllib/Logic and Bit Operations/Bit Slice  Commented=on  lidx=7  ridx=0
  Constant1 : Constant  Commented=on  Value=255  OutDataTypeStr=uint8
  Constant2 : Constant  Commented=on  Value=255  OutDataTypeStr=uint8
  Delay{1,3..9} (8 alike) : Delay  Commented=on  DelayLength=1  InitialCondition=0
  Delay2 : Delay  DelayLength=4  InitialCondition=0
  Display3 : Display  Commented=on
      settings: Format=binary (Stored Integer)
  Divide : Product  Commented=on  Inputs=*/
  GreaterThanOrEqual : RelationalOperator  OutDataTypeStr=boolean  RndMeth=Simplest  InputSameDT=off
  Max : Constant  Commented=on  Value=215  OutDataTypeStr=uint8
  Max1 : Constant  Value=115  OutDataTypeStr=uint8
  Max2 : Constant  Value=0  OutDataTypeStr=uint8
  Min : Constant  Commented=on  Value=0  OutDataTypeStr=uint8
  Product1 : Product  Commented=on  SaturateOnIntegerOverflow=on
  Shift Arithmetic4 : ArithShift  Commented=on  BitShiftNumber=8  BitShiftDirection=Right
  Subtract : Sum  Commented=on  Inputs=+-  AccumDataTypeStr=uint8
  Subtract1 : Sum  Commented=on  Inputs=+-  OutDataTypeStr=uint8
  Switch : Switch  Commented=on  Criteria=u2 > Threshold  SaturateOnIntegerOverflow=off  InputSameDT=off
  Switch1 : Switch  Criteria=u2 > Threshold  SaturateOnIntegerOverflow=off  InputSameDT=off
  Video_out : Outport  OutDataTypeStr=uint8  InitialOutput=[0]
  wires:
  Delay2/1 -> Video_out/1
  Switch1/1 -> Delay2/1
  Max2/1 -> Switch1/3
  GreaterThanOrEqual/1 -> Switch1/2
  channel_in/1 -> GreaterThanOrEqual/1, Switch1/1
  Max1/1 -> GreaterThanOrEqual/2
  Bit Slice/1 -> Switch/3
  Constant1/1 -> Switch/1
  Switch/1 -> Delay1/1
  Shift Arithmetic4/1 -> Switch/2
  Delay9/1 -> Product1/1
  Delay8/1 -> Product1/2
  Delay7/1 -> Subtract1/1
  Delay6/1 -> Subtract1/2
  Delay5/1 -> Divide/2
  Delay4/1 -> Divide/1
  Delay3/1 -> Display3/1, Shift Arithmetic4/1, Bit Slice/1
  Divide/1 -> Delay3/1
  Subtract1/1 -> Delay5/1
  Min/1 -> Subtract/2, Delay6/1
  Max/1 -> Delay7/1
  Product1/1 -> Delay4/1
  Subtract/1 -> Delay8/1
  Constant2/1 -> Delay9/1

== system gm_sobelFilter2024a/sobel_horz_conv_core/Subsystem1 ==
  note: slice out gray
  channel_in : Inport  OutDataTypeStr=uint8
  coeffs : Inport  Port=2
  Enable : EnablePort
  Delay1 : Delay  DelayLength=1  InitialCondition=0
  Delay2 : Delay  DelayLength=1  InitialCondition=0
  Display : Display
      settings: Format=hex (Stored Integer)
  Mux : Mux  Inputs=9
  Product : Product  SaturateOnIntegerOverflow=on
  Sum of Elements : Sum  Inputs=+  OutDataTypeStr=uint8  SaturateOnIntegerOverflow=on
  slicer : Subsystem
  Video_out : Outport  OutDataTypeStr=uint8  InitialOutput=[0]
  wires:
  Delay2/1 -> Video_out/1
  Sum of Elements/1 -> Delay2/1
  Delay1/1 -> Sum of Elements/1
  Product/1 -> Delay1/1
  coeffs/1 -> Display/1, Product/1
  Mux/1 -> Product/2
  slicer/8(out_8) -> Mux/8
  channel_in/1 -> slicer/1(channel_in)
  slicer/2(out_2) -> Mux/2
  slicer/4(out_4) -> Mux/4
  slicer/6(out_6) -> Mux/6
  slicer/3(out_3) -> Mux/3
  slicer/7(out_7) -> Mux/7
  slicer/5(out_5) -> Mux/5
  slicer/9(out_9) -> Mux/9
  slicer/1(out_1) -> Mux/1

== system gm_sobelFilter2024a/sobel_horz_conv_core_alt/Subsystem1 ==
  note: slice out gray
  channel_in : Inport  OutDataTypeStr=uint8
  coeffs : Inport  Port=2
  Enable : EnablePort
  Delay1 : Delay  DelayLength=1  InitialCondition=0
  Delay2 : Delay  DelayLength=1  InitialCondition=0
  Display : Display
      settings: Format=hex (Stored Integer)
  Mux : Mux  Inputs=9
  Product : Product  SaturateOnIntegerOverflow=on
  Sum of Elements : Sum  Inputs=+  OutDataTypeStr=uint8  SaturateOnIntegerOverflow=on
  slicer : Subsystem
  Video_out : Outport  OutDataTypeStr=uint8  InitialOutput=[0]
  wires:
  Delay2/1 -> Video_out/1
  Sum of Elements/1 -> Delay2/1
  Delay1/1 -> Sum of Elements/1
  Product/1 -> Delay1/1
  coeffs/1 -> Display/1, Product/1
  Mux/1 -> Product/2
  slicer/8(out_8) -> Mux/8
  channel_in/1 -> slicer/1(channel_in)
  slicer/2(out_2) -> Mux/2
  slicer/4(out_4) -> Mux/4
  slicer/6(out_6) -> Mux/6
  slicer/3(out_3) -> Mux/3
  slicer/7(out_7) -> Mux/7
  slicer/5(out_5) -> Mux/5
  slicer/9(out_9) -> Mux/9
  slicer/1(out_1) -> Mux/1

== system gm_sobelFilter2024a/sobel_vert_conv_core/Subsystem1 ==
  note: slice out gray
  channel_in : Inport  OutDataTypeStr=uint8
  coeffs : Inport  Port=2
  Enable : EnablePort
  Delay1 : Delay  DelayLength=1  InitialCondition=0
  Delay2 : Delay  DelayLength=1  InitialCondition=0
  Display : Display
      settings: Format=hex (Stored Integer)
  Mux : Mux  Inputs=9
  Product : Product  SaturateOnIntegerOverflow=on
  Sum of Elements : Sum  Inputs=+  OutDataTypeStr=uint8  SaturateOnIntegerOverflow=on
  slicer : Subsystem
  Video_out : Outport  OutDataTypeStr=uint8  InitialOutput=[0]
  wires:
  Delay2/1 -> Video_out/1
  Sum of Elements/1 -> Delay2/1
  Delay1/1 -> Sum of Elements/1
  Product/1 -> Delay1/1
  coeffs/1 -> Display/1, Product/1
  Mux/1 -> Product/2
  slicer/8(out_8) -> Mux/8
  channel_in/1 -> slicer/1(channel_in)
  slicer/2(out_2) -> Mux/2
  slicer/4(out_4) -> Mux/4
  slicer/6(out_6) -> Mux/6
  slicer/3(out_3) -> Mux/3
  slicer/7(out_7) -> Mux/7
  slicer/5(out_5) -> Mux/5
  slicer/9(out_9) -> Mux/9
  slicer/1(out_1) -> Mux/1

== system gm_sobelFilter2024a/sobel_vert_conv_core_alt/Subsystem1 ==
  note: slice out gray
  channel_in : Inport  OutDataTypeStr=uint8
  coeffs : Inport  Port=2
  Enable : EnablePort
  Delay1 : Delay  DelayLength=1  InitialCondition=0
  Delay2 : Delay  DelayLength=1  InitialCondition=0
  Display : Display
      settings: Format=hex (Stored Integer)
  Mux : Mux  Inputs=9
  Product : Product  SaturateOnIntegerOverflow=on
  Sum of Elements : Sum  Inputs=+  OutDataTypeStr=uint8  SaturateOnIntegerOverflow=on
  slicer : Subsystem
  Video_out : Outport  OutDataTypeStr=uint8  InitialOutput=[0]
  wires:
  Delay2/1 -> Video_out/1
  Sum of Elements/1 -> Delay2/1
  Delay1/1 -> Sum of Elements/1
  Product/1 -> Delay1/1
  coeffs/1 -> Display/1, Product/1
  Mux/1 -> Product/2
  slicer/8(out_8) -> Mux/8
  channel_in/1 -> slicer/1(channel_in)
  slicer/2(out_2) -> Mux/2
  slicer/4(out_4) -> Mux/4
  slicer/6(out_6) -> Mux/6
  slicer/3(out_3) -> Mux/3
  slicer/7(out_7) -> Mux/7
  slicer/5(out_5) -> Mux/5
  slicer/9(out_9) -> Mux/9
  slicer/1(out_1) -> Mux/1

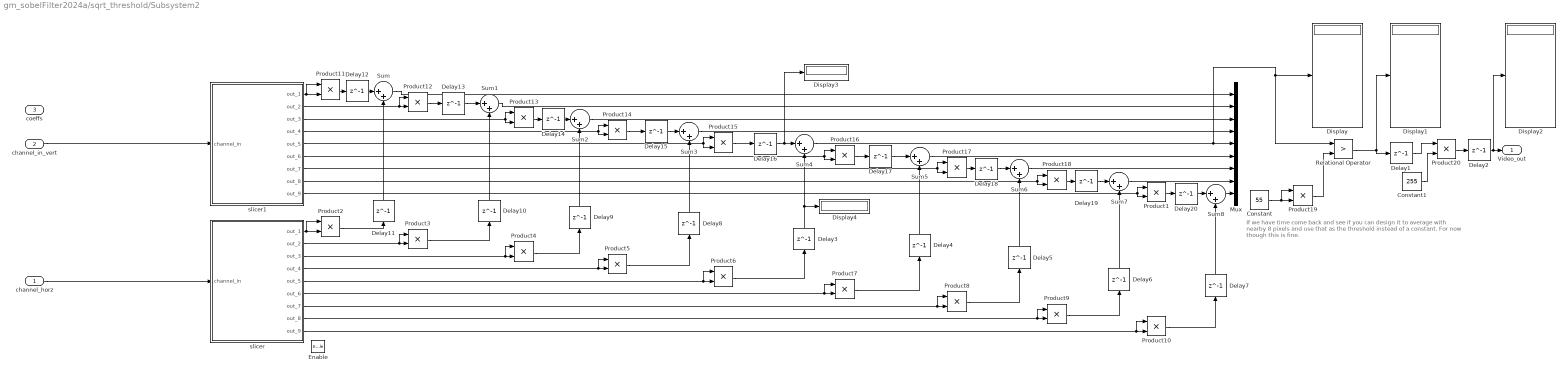
== system gm_sobelFilter2024a/sqrt_threshold/Subsystem2 ==
  note: If we have time come back and see if you can design it to average with
      | nearby 8 pixels and use that as the threshold instead of a constant. For
      |  now though this is fine.
  channel_horz : Inport  OutDataTypeStr=uint8
  channel_in_vert : Inport  Port=2
  coeffs : Inport  Port=3
  Enable : EnablePort
  Constant : Constant  Value=55  OutDataTypeStr=uint8
  Constant1 : Constant  Value=255  OutDataTypeStr=uint8
  Delay{1..20} (20 alike) : Delay  DelayLength=1  InitialCondition=0
  Display{,1..4} (5 alike) : Display
      settings: Format=decimal (Stored Integer)
  Mux : Mux  Inputs=9
  Product{1..20} (20 alike) : Product  SaturateOnIntegerOverflow=on
  Relational Operator : RelationalOperator  Operator=>  OutDataTypeStr=boolean  InputSameDT=off
  Sum{,1..8} (9 alike) : Sum  Inputs=|++
  slicer : Subsystem
  slicer1 : Subsystem
  Video_out : Outport  OutDataTypeStr=uint8  InitialOutput=[0]
  wires:
  Product20/1 -> Delay2/1
  Constant1/1 -> Product20/2
  Sum4/1 -> Mux/5, Relational Operator/1, Display/1
  Relational Operator/1 -> Delay1/1, Display1/1
  Product19/1 -> Relational Operator/2
  Constant/1 -> Product19/2, Product19/1
  Sum/1 -> Mux/1
  Sum1/1 -> Mux/2
  Sum2/1 -> Mux/3
  Sum3/1 -> Mux/4
  Sum5/1 -> Mux/6
  Sum6/1 -> Mux/7
  Sum7/1 -> Mux/8
  Sum8/1 -> Mux/9
  Delay20/1 -> Sum8/1
  Product1/1 -> Delay20/1
  Delay19/1 -> Sum7/1
  Product18/1 -> Delay19/1
  Delay18/1 -> Sum6/1
  Product17/1 -> Delay18/1
  Delay17/1 -> Sum5/1
  Delay16/1 -> Sum4/1, Display3/1
  Delay15/1 -> Sum3/1
  Delay14/1 -> Sum2/1
  Product13/1 -> Delay14/1
  Delay13/1 -> Sum1/1
  Delay12/1 -> Sum/1
  Product11/1 -> Delay12/1
  Delay11/1 -> Sum/2
  Delay10/1 -> Sum1/2
  Delay9/1 -> Sum2/2
  Delay8/1 -> Sum3/2
  Delay7/1 -> Sum8/2
  Delay6/1 -> Sum7/2
  Delay5/1 -> Sum6/2
  Delay4/1 -> Sum5/2
  Delay3/1 -> Sum4/2, Display4/1
  Delay1/1 -> Product20/1
  Product10/1 -> Delay7/1
  Product9/1 -> Delay6/1
  Product8/1 -> Delay5/1
  Product7/1 -> Delay4/1
  Product16/1 -> Delay17/1
  Product6/1 -> Delay3/1
  Product15/1 -> Delay16/1
  Product5/1 -> Delay8/1
  Product14/1 -> Delay15/1
  Product4/1 -> Delay9/1
  Product3/1 -> Delay10/1
  Product12/1 -> Delay13/1
  Product2/1 -> Delay11/1
  channel_in_vert/1 -> slicer1/1(channel_in)
  slicer1/4(out_4) -> Product14/1, Product14/2
  slicer1/6(out_6) -> Product16/1, Product16/2
  slicer1/5(out_5) -> Product15/1, Product15/2
  slicer1/7(out_7) -> Product17/1, Product17/2
  slicer1/3(out_3) -> Product13/1, Product13/2
  slicer1/1(out_1) -> Product11/2, Product11/1
  slicer1/9(out_9) -> Product1/1, Product1/2
  slicer1/2(out_2) -> Product12/2, Product12/1
  slicer1/8(out_8) -> Product18/1, Product18/2
  slicer/9(out_9) -> Product10/2, Product10/1
  Delay2/1 -> Video_out/1, Display2/1
  slicer/8(out_8) -> Product9/2, Product9/1
  channel_horz/1 -> slicer/1(channel_in)
  slicer/2(out_2) -> Product3/2, Product3/1
  slicer/4(out_4) -> Product5/2, Product5/1
  slicer/6(out_6) -> Product7/2, Product7/1
  slicer/3(out_3) -> Product4/2, Product4/1
  slicer/7(out_7) -> Product8/2, Product8/1
  slicer/5(out_5) -> Product6/2, Product6/1
  slicer/1(out_1) -> Product2/2, Product2/1

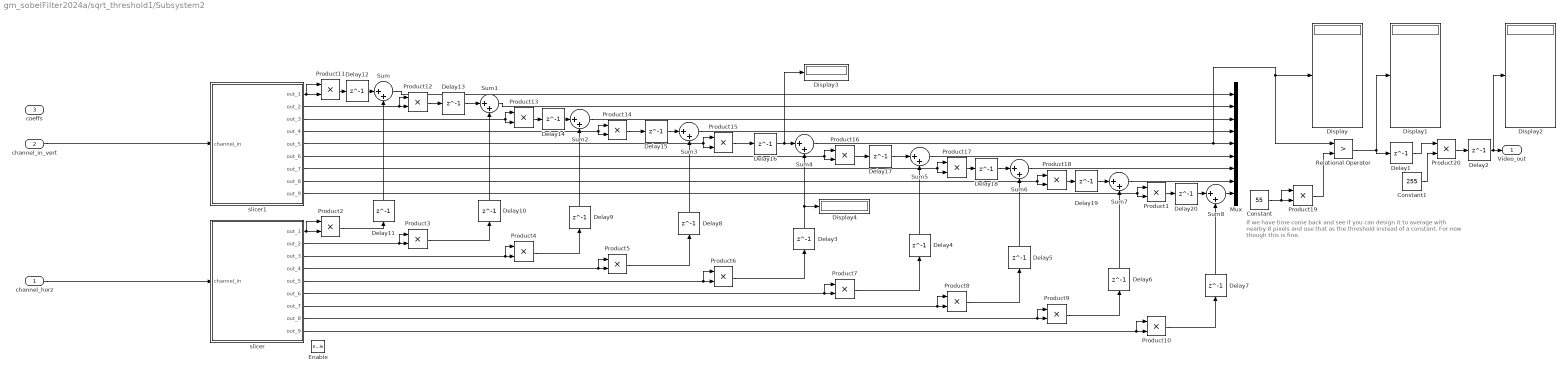
== system gm_sobelFilter2024a/sqrt_threshold1/Subsystem2 ==
  note: If we have time come back and see if you can design it to average with
      | nearby 8 pixels and use that as the threshold instead of a constant. For
      |  now though this is fine.
  channel_horz : Inport  OutDataTypeStr=uint8
  channel_in_vert : Inport  Port=2
  coeffs : Inport  Port=3
  Enable : EnablePort
  Constant : Constant  Value=55  OutDataTypeStr=uint8
  Constant1 : Constant  Value=255  OutDataTypeStr=uint8
  Delay{1..20} (20 alike) : Delay  DelayLength=1  InitialCondition=0
  Display{,1..4} (5 alike) : Display
      settings: Format=decimal (Stored Integer)
  Mux : Mux  Inputs=9
  Product{1..20} (20 alike) : Product  SaturateOnIntegerOverflow=on
  Relational Operator : RelationalOperator  Operator=>  OutDataTypeStr=boolean  InputSameDT=off
  Sum{,1..8} (9 alike) : Sum  Inputs=|++
  slicer : Subsystem
  slicer1 : Subsystem
  Video_out : Outport  OutDataTypeStr=uint8  InitialOutput=[0]
  wires:
  Product20/1 -> Delay2/1
  Constant1/1 -> Product20/2
  Sum4/1 -> Mux/5, Relational Operator/1, Display/1
  Relational Operator/1 -> Delay1/1, Display1/1
  Product19/1 -> Relational Operator/2
  Constant/1 -> Product19/2, Product19/1
  Sum/1 -> Mux/1
  Sum1/1 -> Mux/2
  Sum2/1 -> Mux/3
  Sum3/1 -> Mux/4
  Sum5/1 -> Mux/6
  Sum6/1 -> Mux/7
  Sum7/1 -> Mux/8
  Sum8/1 -> Mux/9
  Delay20/1 -> Sum8/1
  Product1/1 -> Delay20/1
  Delay19/1 -> Sum7/1
  Product18/1 -> Delay19/1
  Delay18/1 -> Sum6/1
  Product17/1 -> Delay18/1
  Delay17/1 -> Sum5/1
  Delay16/1 -> Sum4/1, Display3/1
  Delay15/1 -> Sum3/1
  Delay14/1 -> Sum2/1
  Product13/1 -> Delay14/1
  Delay13/1 -> Sum1/1
  Delay12/1 -> Sum/1
  Product11/1 -> Delay12/1
  Delay11/1 -> Sum/2
  Delay10/1 -> Sum1/2
  Delay9/1 -> Sum2/2
  Delay8/1 -> Sum3/2
  Delay7/1 -> Sum8/2
  Delay6/1 -> Sum7/2
  Delay5/1 -> Sum6/2
  Delay4/1 -> Sum5/2
  Delay3/1 -> Sum4/2, Display4/1
  Delay1/1 -> Product20/1
  Product10/1 -> Delay7/1
  Product9/1 -> Delay6/1
  Product8/1 -> Delay5/1
  Product7/1 -> Delay4/1
  Product16/1 -> Delay17/1
  Product6/1 -> Delay3/1
  Product15/1 -> Delay16/1
  Product5/1 -> Delay8/1
  Product14/1 -> Delay15/1
  Product4/1 -> Delay9/1
  Product3/1 -> Delay10/1
  Product12/1 -> Delay13/1
  Product2/1 -> Delay11/1
  channel_in_vert/1 -> slicer1/1(channel_in)
  slicer1/4(out_4) -> Product14/1, Product14/2
  slicer1/6(out_6) -> Product16/1, Product16/2
  slicer1/5(out_5) -> Product15/1, Product15/2
  slicer1/7(out_7) -> Product17/1, Product17/2
  slicer1/3(out_3) -> Product13/1, Product13/2
  slicer1/1(out_1) -> Product11/2, Product11/1
  slicer1/9(out_9) -> Product1/1, Product1/2
  slicer1/2(out_2) -> Product12/2, Product12/1
  slicer1/8(out_8) -> Product18/1, Product18/2
  slicer/9(out_9) -> Product10/2, Product10/1
  Delay2/1 -> Video_out/1, Display2/1
  slicer/8(out_8) -> Product9/2, Product9/1
  channel_horz/1 -> slicer/1(channel_in)
  slicer/2(out_2) -> Product3/2, Product3/1
  slicer/4(out_4) -> Product5/2, Product5/1
  slicer/6(out_6) -> Product7/2, Product7/1
  slicer/3(out_3) -> Product4/2, Product4/1
  slicer/7(out_7) -> Product8/2, Product8/1
  slicer/5(out_5) -> Product6/2, Product6/1
  slicer/1(out_1) -> Product2/2, Product2/1

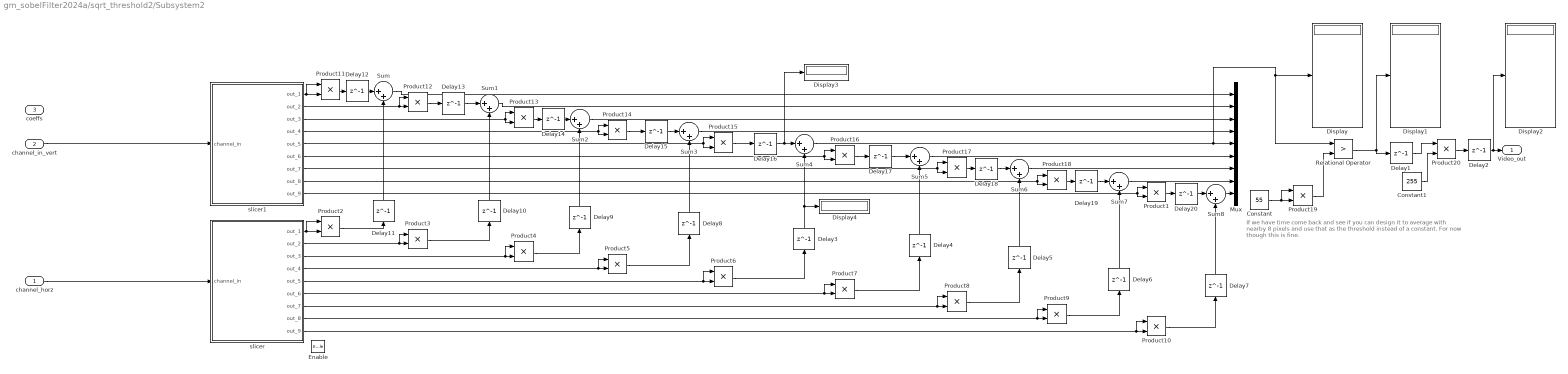
== system gm_sobelFilter2024a/sqrt_threshold2/Subsystem2 ==
  note: If we have time come back and see if you can design it to average with
      | nearby 8 pixels and use that as the threshold instead of a constant. For
      |  now though this is fine.
  channel_horz : Inport  OutDataTypeStr=uint8
  channel_in_vert : Inport  Port=2
  coeffs : Inport  Port=3
  Enable : EnablePort
  Constant : Constant  Value=55  OutDataTypeStr=uint8
  Constant1 : Constant  Value=255  OutDataTypeStr=uint8
  Delay{1..20} (20 alike) : Delay  DelayLength=1  InitialCondition=0
  Display{,1..4} (5 alike) : Display
      settings: Format=decimal (Stored Integer)
  Mux : Mux  Inputs=9
  Product{1..20} (20 alike) : Product  SaturateOnIntegerOverflow=on
  Relational Operator : RelationalOperator  Operator=>  OutDataTypeStr=boolean  InputSameDT=off
  Sum{,1..8} (9 alike) : Sum  Inputs=|++
  slicer : Subsystem
  slicer1 : Subsystem
  Video_out : Outport  OutDataTypeStr=uint8  InitialOutput=[0]
  wires:
  Product20/1 -> Delay2/1
  Constant1/1 -> Product20/2
  Sum4/1 -> Mux/5, Relational Operator/1, Display/1
  Relational Operator/1 -> Delay1/1, Display1/1
  Product19/1 -> Relational Operator/2
  Constant/1 -> Product19/2, Product19/1
  Sum/1 -> Mux/1
  Sum1/1 -> Mux/2
  Sum2/1 -> Mux/3
  Sum3/1 -> Mux/4
  Sum5/1 -> Mux/6
  Sum6/1 -> Mux/7
  Sum7/1 -> Mux/8
  Sum8/1 -> Mux/9
  Delay20/1 -> Sum8/1
  Product1/1 -> Delay20/1
  Delay19/1 -> Sum7/1
  Product18/1 -> Delay19/1
  Delay18/1 -> Sum6/1
  Product17/1 -> Delay18/1
  Delay17/1 -> Sum5/1
  Delay16/1 -> Sum4/1, Display3/1
  Delay15/1 -> Sum3/1
  Delay14/1 -> Sum2/1
  Product13/1 -> Delay14/1
  Delay13/1 -> Sum1/1
  Delay12/1 -> Sum/1
  Product11/1 -> Delay12/1
  Delay11/1 -> Sum/2
  Delay10/1 -> Sum1/2
  Delay9/1 -> Sum2/2
  Delay8/1 -> Sum3/2
  Delay7/1 -> Sum8/2
  Delay6/1 -> Sum7/2
  Delay5/1 -> Sum6/2
  Delay4/1 -> Sum5/2
  Delay3/1 -> Sum4/2, Display4/1
  Delay1/1 -> Product20/1
  Product10/1 -> Delay7/1
  Product9/1 -> Delay6/1
  Product8/1 -> Delay5/1
  Product7/1 -> Delay4/1
  Product16/1 -> Delay17/1
  Product6/1 -> Delay3/1
  Product15/1 -> Delay16/1
  Product5/1 -> Delay8/1
  Product14/1 -> Delay15/1
  Product4/1 -> Delay9/1
  Product3/1 -> Delay10/1
  Product12/1 -> Delay13/1
  Product2/1 -> Delay11/1
  channel_in_vert/1 -> slicer1/1(channel_in)
  slicer1/4(out_4) -> Product14/1, Product14/2
  slicer1/6(out_6) -> Product16/1, Product16/2
  slicer1/5(out_5) -> Product15/1, Product15/2
  slicer1/7(out_7) -> Product17/1, Product17/2
  slicer1/3(out_3) -> Product13/1, Product13/2
  slicer1/1(out_1) -> Product11/2, Product11/1
  slicer1/9(out_9) -> Product1/1, Product1/2
  slicer1/2(out_2) -> Product12/2, Product12/1
  slicer1/8(out_8) -> Product18/1, Product18/2
  slicer/9(out_9) -> Product10/2, Product10/1
  Delay2/1 -> Video_out/1, Display2/1
  slicer/8(out_8) -> Product9/2, Product9/1
  channel_horz/1 -> slicer/1(channel_in)
  slicer/2(out_2) -> Product3/2, Product3/1
  slicer/4(out_4) -> Product5/2, Product5/1
  slicer/6(out_6) -> Product7/2, Product7/1
  slicer/3(out_3) -> Product4/2, Product4/1
  slicer/7(out_7) -> Product8/2, Product8/1
  slicer/5(out_5) -> Product6/2, Product6/1
  slicer/1(out_1) -> Product2/2, Product2/1
